simulink model "VisionModel_v7"  (Simulink 7.6)
settings: Solver=FixedStepDiscrete  StartTime=0.0  StopTime=0  RelTol=1e-3
values from neighbouring files (symbols this model uses):
  Down_Camera_Dimensions = [120 160]    [VisionConstants.m]
  Forward_Camera_Dimensions = [160 120]    [VisionConstants.m]
  Iter_Segment_Thresh = 60    [VisionConstants.m]
  Scale_Down_B = 1    [VisionConstants.m]
  Scale_Down_G = 1    [VisionConstants.m]
  Scale_Down_H = 1    [VisionConstants.m]
  Scale_Down_R = 1    [VisionConstants.m]
  Scale_Down_S = 1    [VisionConstants.m]
  Scale_Down_V = 5    [VisionConstants.m]
  Scale_Forward_B = 0    [VisionConstants.m]
  Scale_Forward_G = 1    [VisionConstants.m]
  Scale_Forward_H = 1    [VisionConstants.m]
  Scale_Forward_R = 0    [VisionConstants.m]
  Scale_Forward_S = 1    [VisionConstants.m]
  Scale_Forward_V = 5    [VisionConstants.m]
undefined symbols (not defined in the file or in its folder): Forward_Fov, Rec, SDTV
libraries: vipconversions x6, vipgeotforms x3, vipanalysis x2, viptransforms x2, viptextngfix x2
(part 1 of 2)
settings Model: Creator=Administrator  LastModifiedBy=auvt
settings OptimizationCC: OptimizeModelRefInitCode=on
settings RTWCC: SystemTargetFile=ert.tlc  GenCodeOnly=on  TemplateMakefile=ert_default_tmf  PostCodeGenCommand=packNGo(buildInfo, {'packType' 'flat'})  Description=Real-Time Workshop Embedded Coder  GenerateReport=on  ProcessScript=ert_make_rtw_hook  IncludeHyperlinkInReport=on  LaunchReport=on  TargetLang=C++
settings CodeAppCC: IgnoreCustomStorageClasses=off
settings ERTTargetCC: MultiwordLength=2048  GenerateSampleERTMain=on  IncludeMdlTerminateFcn=off  ERTCustomFileTemplate=example_file_process.tlc  ConvertIfToSwitch=off

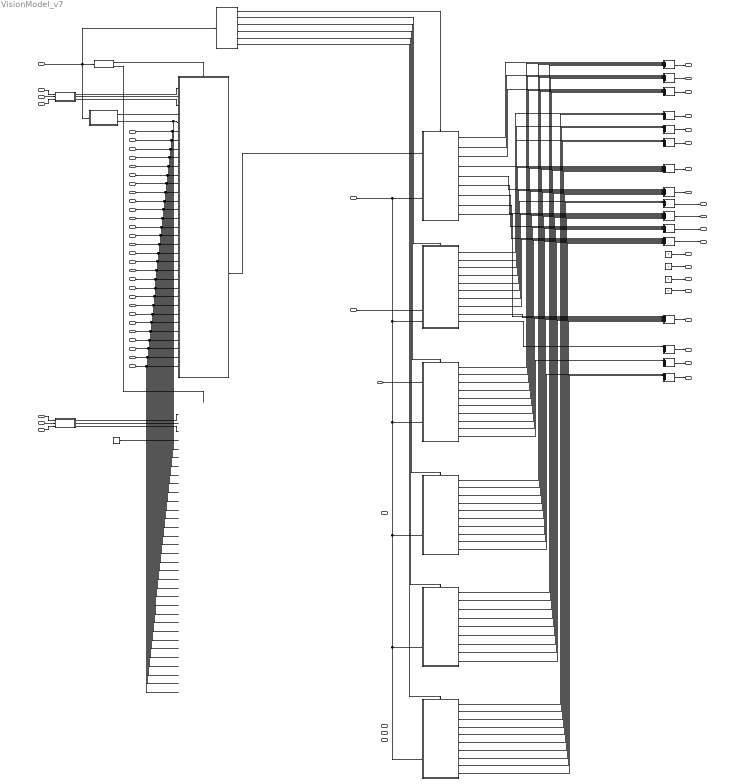
== system VisionModel_v7 ==
  note: Forward camera QImage array
  note: Down camera QImage array
  note: Forward
  note: Down
  note: Current target information
  note: Desired target information
  note: Mode and general target information
  note: Note: TargetFound, and the last three inputs to MotionController.mdl,
      | can be changed by the script, not the vision model.
  note: Path-following variables
      | DesiredPathDirection:
      | 0 = Use internal default
      | 1 = Take left path
      | 2 = Take right path
  note: Drop mechanism variables
  R_forward_in : Inport  PortDimensions=Forward_Camera_Dimensions
  G_forward_in : Inport  Port=2  PortDimensions=Forward_Camera_Dimensions
  B_forward_in : Inport  Port=3  PortDimensions=Forward_Camera_Dimensions
  R_down_in : Inport  Port=4  PortDimensions=Down_Camera_Dimensions
  G_down_in : Inport  Port=5  PortDimensions=Down_Camera_Dimensions
  B_down_in : Inport  Port=6  PortDimensions=Down_Camera_Dimensions
  ModeSelect : Inport  Port=7
  OutputImage : Inport  Port=8
  DesiredPathDirection : Inport  Port=9
  DesiredBuoyColor : Inport  Port=10
  DesiredTorpedoColor : Inport  Port=11
  ProceedToSecondTarget : Inport  Port=12
  DefaultTargetShape : Inport  Port=13
  DefaultTargetColor : Inport  Port=14
  white_al : Inport  Port=15
  white_au : Inport  Port=16
  white_bl : Inport  Port=17
  white_bu : Inport  Port=18
  black_al : Inport  Port=19
  black_au : Inport  Port=20
  black_bl : Inport  Port=21
  black_bu : Inport  Port=22
  blue_al : Inport  Port=23
  blue_au : Inport  Port=24
  blue_bl : Inport  Port=25
  blue_bu : Inport  Port=26
  red_al : Inport  Port=27
  red_au : Inport  Port=28
  red_bl : Inport  Port=29
  red_bu : Inport  Port=30
  orange_al : Inport  Port=31
  orane_au : Inport  Port=32
  orange_bl : Inport  Port=33
  orange_bu : Inport  Port=34
  yellow_al : Inport  Port=35
  yellow_au : Inport  Port=36
  yellow_bl : Inport  Port=37
  yellow_bu : Inport  Port=38
  green_al : Inport  Port=39
  green_au : Inport  Port=40
  breen_bl : Inport  Port=41
  green_bu : Inport  Port=42
  Add{,2..6,18..27} (16 alike) : Sum  Inputs=++++++
  Blob_Analysis : Subsystem  TreatAsAtomicUnit=on
  ColorSelect : Subsystem  TreatAsAtomicUnit=on
  Constant{,1..3} (4 alike) : Constant  Value=0
  Down Filter : Subsystem
  Forward Filter : Subsystem
  If1 : If  IfExpression=u1 == 1 | u1 == 3 | u1 == 4 | u1 == 5  ElseIfExpressions=u1 == 2 | u1 == 6  ShowElse=off
  If2 : If  IfExpression=u1 == 1  ElseIfExpressions=u1 == 2, u1 == 3, u1 == 4, u1 == 5, u1 == 6  ShowElse=off
  L_detector : Subsystem  TreatAsAtomicUnit=on
  ModeSelect1 : Constant  Value=[2 0 0 0 0 0 0 0 0 0]  SampleTime=-1
  buoy_detector : Subsystem  TreatAsAtomicUnit=on
  drop_mech : Subsystem  TreatAsAtomicUnit=on
  path_detector : Subsystem  TreatAsAtomicUnit=on
  torpedo : Subsystem  TreatAsAtomicUnit=on
  validation_gate : Subsystem  TreatAsAtomicUnit=on
  R_forward_out : Outport  OutDataTypeStr=double
  G_forward_out : Outport  Port=2  OutDataTypeStr=double
  B_forward_out : Outport  Port=3  OutDataTypeStr=double
  R_down_out : Outport  Port=4  OutDataTypeStr=double
  G_down_out : Outport  Port=5  OutDataTypeStr=double
  B_down_out : Outport  Port=6  OutDataTypeStr=double
  TargetSelect : Outport  Port=7  OutDataTypeStr=double
  MaintainHeading : Outport  Port=8  OutDataTypeStr=double
  TargetX : Outport  Port=9  OutDataTypeStr=double
  TargetY : Outport  Port=10  OutDataTypeStr=double
  TargetZ : Outport  Port=11  OutDataTypeStr=double
  TargetYaw : Outport  Port=12  OutDataTypeStr=double
  DesiredTargetX : Outport  Port=13  OutDataTypeStr=double
  DesiredTargetY : Outport  Port=14  OutDataTypeStr=double
  DesiredTargetZ : Outport  Port=15  OutDataTypeStr=double
  DesiredTargetYaw : Outport  Port=16  OutDataTypeStr=double
  TargetDetected : Outport  Port=17  OutDataTypeStr=double
  PathState : Outport  Port=18  OutDataTypeStr=double
  BuoyColors : Outport  Port=19  OutDataTypeStr=double
  FireAuthorization : Outport  Port=20  OutDataTypeStr=double
  wires:
  G_down_in/1 -> Down Filter/2(G_in)
  R_down_in/1 -> Down Filter/1(R_in)
  B_down_in/1 -> Down Filter/3(B_in)
  If1/1 -> Blob_Analysis/Action
  If1/2 -> ?
  R_forward_in/1 -> Forward Filter/1(R_in)
  Forward Filter/2(G_out) -> Blob_Analysis/2(G_in)
  Forward Filter/1(R_out) -> Blob_Analysis/1(R_in)
  Forward Filter/3(B_out) -> Blob_Analysis/3(B_in)
  G_forward_in/1 -> Forward Filter/2(G_in)
  B_forward_in/1 -> Forward Filter/3(B_in)
  Down Filter/2(G_out) -> ?
  Down Filter/1(R_out) -> ?
  Down Filter/3(B_out) -> ?
  Blob_Analysis/11(bw_image) -> validation_gate/1(bw_image)
  white_al/1 -> Blob_Analysis/6(white_al)
  white_au/1 -> Blob_Analysis/7(white_au)
  white_bl/1 -> Blob_Analysis/8(white_bl)
  white_bu/1 -> Blob_Analysis/9(white_bu)
  black_al/1 -> Blob_Analysis/10(black_al)
  black_au/1 -> Blob_Analysis/11(black_au)
  black_bl/1 -> Blob_Analysis/12(black_bl)
  black_bu/1 -> Blob_Analysis/13(black_bu)
  blue_al/1 -> Blob_Analysis/14(blue_al)
  blue_au/1 -> Blob_Analysis/15(blue_au)
  blue_bl/1 -> Blob_Analysis/16(blue_bl)
  blue_bu/1 -> Blob_Analysis/17(blue_bu)
  red_al/1 -> Blob_Analysis/18(red_al)
  red_au/1 -> Blob_Analysis/19(red_au)
  red_bl/1 -> Blob_Analysis/20(red_bl)
  red_bu/1 -> Blob_Analysis/21(red_bu)
  orange_al/1 -> Blob_Analysis/22(orange_al)
  orane_au/1 -> Blob_Analysis/23(orane_au)
  orange_bl/1 -> Blob_Analysis/24(orange_bl)
  orange_bu/1 -> Blob_Analysis/25(orange_bu)
  yellow_al/1 -> Blob_Analysis/26(yellow_al)
  yellow_au/1 -> Blob_Analysis/27(yellow_au)
  yellow_bl/1 -> Blob_Analysis/28(yellow_bl)
  yellow_bu/1 -> Blob_Analysis/29(yellow_bu)
  green_al/1 -> Blob_Analysis/30(green_al)
  green_au/1 -> Blob_Analysis/31(green_au)
  breen_bl/1 -> Blob_Analysis/32(breen_bl)
  green_bu/1 -> Blob_Analysis/33(green_bu)
  If2/1 -> validation_gate/Action
  Add2/1 -> MaintainHeading/1
  Add3/1 -> TargetX/1
  Add4/1 -> TargetY/1
  Add5/1 -> TargetZ/1
  Add6/1 -> TargetYaw/1
  Add19/1 -> PathState/1
  Add22/1 -> R_forward_out/1
  Add23/1 -> G_forward_out/1
  Add24/1 -> B_forward_out/1
  Constant/1 -> DesiredTargetX/1
  Constant3/1 -> DesiredTargetYaw/1
  Constant2/1 -> DesiredTargetZ/1
  Constant1/1 -> DesiredTargetY/1
  Add20/1 -> BuoyColors/1
  Add21/1 -> FireAuthorization/1
  validation_gate/1(R_forward_out) -> Add22/1
  validation_gate/2(G_forward_out) -> Add23/1
  validation_gate/3(B_forward_out) -> Add24/1
  validation_gate/4(TargetSelect) -> Add/1
  validation_gate/5(MaintainHeading) -> Add2/1
  validation_gate/6(TargetY) -> Add4/1
  validation_gate/7(TargetZ) -> Add5/1
  validation_gate/8(TargetYaw) -> Add6/1
  validation_gate/9(TargetDetected) -> Add18/1
  path_detector/1(R_down_out) -> Add25/1
  path_detector/2(G_down_out) -> Add26/1
  path_detector/3(B_down_out) -> Add27/1
  path_detector/4(TargetSelect) -> Add/2
  path_detector/5(MaintainHeading) -> Add2/2
  path_detector/6(TargetX) -> Add3/1
  path_detector/7(TargetY) -> Add4/2
  path_detector/8(TargetYaw) -> Add6/2
  path_detector/9(TargetDetected) -> Add18/2
  path_detector/10(PathState) -> Add19/1
  buoy_detector/1(R_forward_out) -> Add22/2
  buoy_detector/2(G_forward_out) -> Add23/2
  buoy_detector/3(B_forward_out) -> Add24/2
  buoy_detector/4(TargetSelect) -> Add/3
  buoy_detector/5(MaintainHeading) -> Add2/3
  buoy_detector/6(TargetY) -> Add4/3
  buoy_detector/7(TargetZ) -> Add5/2
  buoy_detector/8(TargetYaw) -> Add6/3
  buoy_detector/9(TargetDetected) -> Add18/3
  buoy_detector/10(BuoyColors) -> Add20/1
  torpedo/1(R_forward_out) -> Add22/3
  torpedo/2(G_forward_out) -> Add23/3
  torpedo/3(B_forward_out) -> Add24/3
  torpedo/4(TargetSelect) -> Add/4
  torpedo/5(MaintainHeading) -> Add2/4
  torpedo/6(TargetY) -> Add4/4
  torpedo/7(TargetZ) -> Add5/3
  torpedo/8(TargetYaw) -> Add6/4
  torpedo/10(FireAuthorization) -> Add21/1
  torpedo/9(TargetDetected) -> Add18/4
  L_detector/1(R_forward_out) -> Add22/4
  L_detector/2(G_forward_out) -> Add23/4
  L_detector/3(B_forward_out) -> Add24/4
  L_detector/4(TargetSelect) -> Add/5
  L_detector/5(MaintainHeading) -> Add2/5
  L_detector/6(TargetY) -> Add4/5
  L_detector/7(TargetZ) -> Add5/4
  L_detector/8(TargetYaw) -> Add6/5
  L_detector/9(TargetDetected) -> Add18/5
  drop_mech/1(R_down_out) -> Add25/2
  drop_mech/2(G_down_out) -> Add26/2
  drop_mech/3(B_down_out) -> Add27/2
  drop_mech/4(TargetSelect) -> Add/6
  drop_mech/5(MaintainHeading) -> Add2/6
  drop_mech/6(TargetX) -> Add3/2
  drop_mech/7(TargetY) -> Add4/6
  drop_mech/8(TargetYaw) -> Add6/6
  drop_mech/9(TargetDetected) -> Add18/6
  drop_mech/10(FireAuthorization) -> Add21/2
  ModeSelect/1 -> If1/1, ColorSelect/1(ModeSelect), If2/1
  If2/2 -> path_detector/Action
  If2/3 -> buoy_detector/Action
  If2/4 -> torpedo/Action
  If2/5 -> L_detector/Action
  If2/6 -> drop_mech/Action
  ColorSelect/1(ColorFilter) -> Blob_Analysis/4(ColorFilter)
  ColorSelect/2(OutputSegmentedImage) -> Blob_Analysis/5(OutputSegmentedImage)
  OutputImage/1 -> validation_gate/2(output_image), buoy_detector/2(output_image), torpedo/2(output_image), L_detector/2(output_image), drop_mech/2(output_image), path_detector/7(output_image)
  DesiredBuoyColor/1 -> buoy_detector/1(DesiredBuoyColor)
  DesiredPathDirection/1 -> path_detector/6(DesiredPathDirection)
  ? -> path_detector/1(bw_image)
  ? -> path_detector/2(blob_count)
  ? -> path_detector/3(blob_area)
  ? -> path_detector/4(blob_centroids)
  ? -> path_detector/5(blob_orientation)
  ModeSelect1/1 -> ?
  Add/1 -> TargetSelect/1
  Add25/1 -> R_down_out/1
  Add26/1 -> G_down_out/1
  Add27/1 -> B_down_out/1
  Add18/1 -> TargetDetected/1

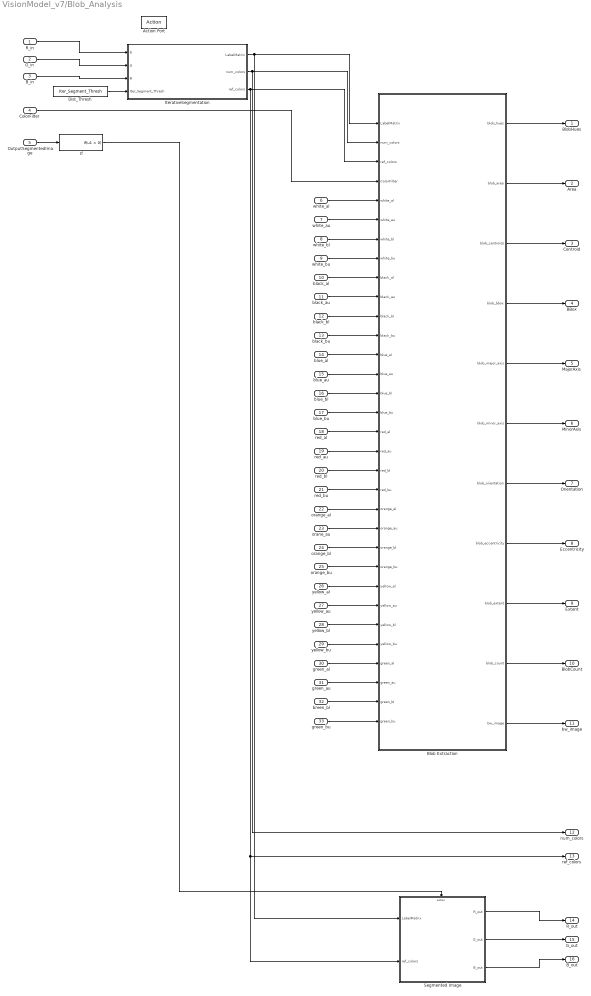
== system VisionModel_v7/Blob_Analysis ==
  R_in : Inport
  G_in : Inport  Port=2
  B_in : Inport  Port=3
  ColorFilter : Inport  Port=4
  OutputSegmentedImage : Inport  Port=5
  white_al : Inport  Port=6
  white_au : Inport  Port=7
  white_bl : Inport  Port=8
  white_bu : Inport  Port=9
  black_al : Inport  Port=10
  black_au : Inport  Port=11
  black_bl : Inport  Port=12
  black_bu : Inport  Port=13
  blue_al : Inport  Port=14
  blue_au : Inport  Port=15
  blue_bl : Inport  Port=16
  blue_bu : Inport  Port=17
  red_al : Inport  Port=18
  red_au : Inport  Port=19
  red_bl : Inport  Port=20
  red_bu : Inport  Port=21
  orange_al : Inport  Port=22
  orane_au : Inport  Port=23
  orange_bl : Inport  Port=24
  orange_bu : Inport  Port=25
  yellow_al : Inport  Port=26
  yellow_au : Inport  Port=27
  yellow_bl : Inport  Port=28
  yellow_bu : Inport  Port=29
  green_al : Inport  Port=30
  green_au : Inport  Port=31
  breen_bl : Inport  Port=32
  green_bu : Inport  Port=33
  Action Port : ActionPort  ActionType=then
  Blob Extraction : Stateflow chart  TreatAsAtomicUnit=on
  Dist_Thresh : Constant  Value=Iter_Segment_Thresh  SampleTime=-1
  If : If  ShowElse=off
  IterativeSegmentation : Subsystem
      settings: UndoDeleteFcn=Stateflow.SLINSF.SimulinkMan.restorePreDeleteFcn  PreDeleteFcn=Stateflow.SLINSF.SimulinkMan.removePreDeleteFcn
  Segmented Image : Subsystem  TreatAsAtomicUnit=on
  BlobHues : Outport
  Area : Outport  Port=2
  Centroid : Outport  Port=3
  BBox : Outport  Port=4
  MajorAxis : Outport  Port=5
  MinorAxis : Outport  Port=6
  Orientation : Outport  Port=7
  Eccentricity : Outport  Port=8
  Extent : Outport  Port=9
  BlobCount : Outport  Port=10
  bw_image : Outport  Port=11
  num_colors : Outport  Port=12
  ref_colors : Outport  Port=13
  R_out : Outport  Port=14
  G_out : Outport  Port=15
  B_out : Outport  Port=16
  wires:
  Blob Extraction/11(bw_image) -> bw_image/1
  Blob Extraction/10(blob_count) -> BlobCount/1
  Blob Extraction/9(blob_extent) -> Extent/1
  Blob Extraction/8(blob_eccentricity) -> Eccentricity/1
  Blob Extraction/7(blob_orientation) -> Orientation/1
  Blob Extraction/6(blob_minor_axis) -> MinorAxis/1
  Blob Extraction/5(blob_major_axis) -> MajorAxis/1
  Blob Extraction/4(blob_bbox) -> BBox/1
  Blob Extraction/3(blob_centroids) -> Centroid/1
  Blob Extraction/2(blob_area) -> Area/1
  Blob Extraction/1(blob_hues) -> BlobHues/1
  ColorFilter/1 -> Blob Extraction/4(ColorFilter)
  white_al/1 -> Blob Extraction/5(white_al)
  white_au/1 -> Blob Extraction/6(white_au)
  white_bl/1 -> Blob Extraction/7(white_bl)
  white_bu/1 -> Blob Extraction/8(white_bu)
  black_al/1 -> Blob Extraction/9(black_al)
  black_au/1 -> Blob Extraction/10(black_au)
  black_bl/1 -> Blob Extraction/11(black_bl)
  black_bu/1 -> Blob Extraction/12(black_bu)
  blue_au/1 -> Blob Extraction/14(blue_au)
  blue_bl/1 -> Blob Extraction/15(blue_bl)
  blue_bu/1 -> Blob Extraction/16(blue_bu)
  red_al/1 -> Blob Extraction/17(red_al)
  red_au/1 -> Blob Extraction/18(red_au)
  red_bl/1 -> Blob Extraction/19(red_bl)
  red_bu/1 -> Blob Extraction/20(red_bu)
  IterativeSegmentation/1(LabelMatrix) -> Blob Extraction/1(LabelMatrix), Segmented Image/1(LabelMatrix)
  IterativeSegmentation/2(num_colors) -> Blob Extraction/2(num_colors), num_colors/1
  IterativeSegmentation/3(ref_colors) -> Blob Extraction/3(ref_colors), Segmented Image/2(ref_colors), ref_colors/1
  Dist_Thresh/1 -> IterativeSegmentation/4(Iter_Segment_Thresh)
  R_in/1 -> IterativeSegmentation/1(R)
  G_in/1 -> IterativeSegmentation/2(G)
  B_in/1 -> IterativeSegmentation/3(B)
  If/1 -> Segmented Image/Action
  OutputSegmentedImage/1 -> If/1
  Segmented Image/1(R_out) -> R_out/1
  Segmented Image/2(G_out) -> G_out/1
  Segmented Image/3(B_out) -> B_out/1
  green_bu/1 -> Blob Extraction/32(green_bu)
  blue_al/1 -> Blob Extraction/13(blue_al)
  orange_al/1 -> Blob Extraction/21(orange_al)
  orane_au/1 -> Blob Extraction/22(orange_au)
  orange_bl/1 -> Blob Extraction/23(orange_bl)
  orange_bu/1 -> Blob Extraction/24(orange_bu)
  yellow_al/1 -> Blob Extraction/25(yellow_al)
  yellow_au/1 -> Blob Extraction/26(yellow_au)
  yellow_bl/1 -> Blob Extraction/27(yellow_bl)
  yellow_bu/1 -> Blob Extraction/28(yellow_bu)
  green_al/1 -> Blob Extraction/29(green_al)
  green_au/1 -> Blob Extraction/30(green_au)
  breen_bl/1 -> Blob Extraction/31(green_bl)

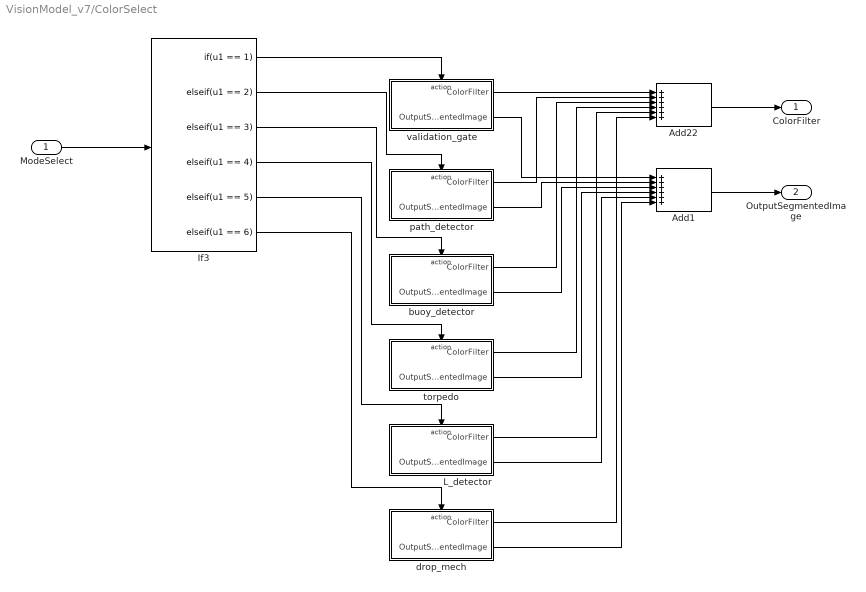
== system VisionModel_v7/ColorSelect ==
  ModeSelect : Inport
  Add1 : Sum  Inputs=++++++
  Add22 : Sum  Inputs=++++++
  If3 : If  IfExpression=u1 == 1  ElseIfExpressions=u1 == 2, u1 == 3, u1 == 4, u1 == 5, u1 == 6  ShowElse=off
  L_detector : Subsystem  TreatAsAtomicUnit=on
  buoy_detector : Subsystem  TreatAsAtomicUnit=on
  drop_mech : Subsystem  TreatAsAtomicUnit=on
  path_detector : Subsystem  TreatAsAtomicUnit=on
  torpedo : Subsystem  TreatAsAtomicUnit=on
  validation_gate : Subsystem  TreatAsAtomicUnit=on
  ColorFilter : Outport  OutDataTypeStr=double
  OutputSegmentedImage : Outport  Port=2  OutDataTypeStr=double
  wires:
  ModeSelect/1 -> If3/1
  If3/1 -> validation_gate/Action
  Add22/1 -> ColorFilter/1
  If3/2 -> path_detector/Action
  If3/3 -> buoy_detector/Action
  If3/4 -> torpedo/Action
  If3/5 -> L_detector/Action
  If3/6 -> drop_mech/Action
  Add1/1 -> OutputSegmentedImage/1
  validation_gate/1(ColorFilter) -> Add22/1
  validation_gate/2(OutputSegmentedImage) -> Add1/1
  path_detector/1(ColorFilter) -> Add22/2
  path_detector/2(OutputSegmentedImage) -> Add1/2
  buoy_detector/1(ColorFilter) -> Add22/3
  buoy_detector/2(OutputSegmentedImage) -> Add1/3
  torpedo/1(ColorFilter) -> Add22/4
  torpedo/2(OutputSegmentedImage) -> Add1/4
  L_detector/1(ColorFilter) -> Add22/5
  L_detector/2(OutputSegmentedImage) -> Add1/5
  drop_mech/1(ColorFilter) -> Add22/6
  drop_mech/2(OutputSegmentedImage) -> Add1/6

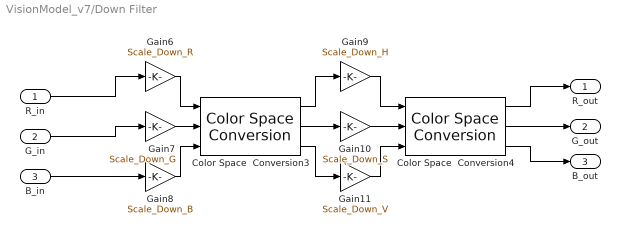
== system VisionModel_v7/Down Filter ==
  R_in : Inport  PortDimensions=Down_Camera_Dimensions
  G_in : Inport  Port=2  PortDimensions=Down_Camera_Dimensions
  B_in : Inport  Port=3  PortDimensions=Down_Camera_Dimensions
  Color Space  Conversion3 : vipconversions/Color Space  Conversion  conversion=Obsolete  conversionActive=R'G'B' to HSV  wp_str=D50  rec=Rec. 601 (SDTV)  sys=1125/60/2:1  imagePorts=Separate color signals
  Color Space  Conversion4 : vipconversions/Color Space  Conversion  conversion=Obsolete  conversionActive=HSV to R'G'B'  wp_str=D50  rec=Rec. 601 (SDTV)  sys=1125/60/2:1  imagePorts=Separate color signals
  Gain10 : Gain  Gain=Scale_Down_S
  Gain11 : Gain  Gain=Scale_Down_V
  Gain6 : Gain  Gain=Scale_Down_R
  Gain7 : Gain  Gain=Scale_Down_G
  Gain8 : Gain  Gain=Scale_Down_B
  Gain9 : Gain  Gain=Scale_Down_H
  R_out : Outport  OutDataTypeStr=double
  G_out : Outport  Port=2  OutDataTypeStr=double
  B_out : Outport  Port=3  OutDataTypeStr=double
  wires:
  Gain6/1 -> Color Space  Conversion3/1
  Gain7/1 -> Color Space  Conversion3/2
  Gain8/1 -> Color Space  Conversion3/3
  Color Space  Conversion3/1 -> Gain9/1
  Color Space  Conversion3/2 -> Gain10/1
  Color Space  Conversion3/3 -> Gain11/1
  Gain9/1 -> Color Space  Conversion4/1
  Gain10/1 -> Color Space  Conversion4/2
  Gain11/1 -> Color Space  Conversion4/3
  R_in/1 -> Gain6/1
  G_in/1 -> Gain7/1
  B_in/1 -> Gain8/1
  Color Space  Conversion4/1 -> R_out/1
  Color Space  Conversion4/2 -> G_out/1
  Color Space  Conversion4/3 -> B_out/1

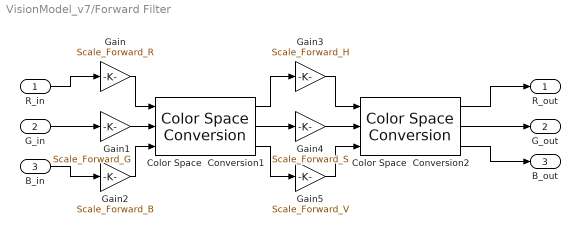
== system VisionModel_v7/Forward Filter ==
  R_in : Inport  PortDimensions=Forward_Camera_Dimensions
  G_in : Inport  Port=2  PortDimensions=Forward_Camera_Dimensions
  B_in : Inport  Port=3  PortDimensions=Forward_Camera_Dimensions
  Color Space  Conversion1 : vipconversions/Color Space  Conversion  conversion=Obsolete  conversionActive=R'G'B' to HSV  wp_str=D50  rec=Rec. 601 (SDTV)  sys=1125/60/2:1  imagePorts=Separate color signals
  Color Space  Conversion2 : vipconversions/Color Space  Conversion  conversion=Obsolete  conversionActive=HSV to R'G'B'  wp_str=D50  rec=Rec. 601 (SDTV)  sys=1125/60/2:1  imagePorts=Separate color signals
  Gain : Gain  Gain=Scale_Forward_R
  Gain1 : Gain  Gain=Scale_Forward_G
  Gain2 : Gain  Gain=Scale_Forward_B
  Gain3 : Gain  Gain=Scale_Forward_H
  Gain4 : Gain  Gain=Scale_Forward_S
  Gain5 : Gain  Gain=Scale_Forward_V
  R_out : Outport  OutDataTypeStr=double
  G_out : Outport  Port=2  OutDataTypeStr=double
  B_out : Outport  Port=3  OutDataTypeStr=double
  wires:
  R_in/1 -> Gain/1
  G_in/1 -> Gain1/1
  B_in/1 -> Gain2/1
  Gain/1 -> Color Space  Conversion1/1
  Gain1/1 -> Color Space  Conversion1/2
  Gain2/1 -> Color Space  Conversion1/3
  Color Space  Conversion1/1 -> Gain3/1
  Color Space  Conversion1/2 -> Gain4/1
  Color Space  Conversion1/3 -> Gain5/1
  Gain3/1 -> Color Space  Conversion2/1
  Gain4/1 -> Color Space  Conversion2/2
  Gain5/1 -> Color Space  Conversion2/3
  Color Space  Conversion2/1 -> R_out/1
  Color Space  Conversion2/2 -> G_out/1
  Color Space  Conversion2/3 -> B_out/1

== system VisionModel_v7/L_detector ==
  bw_image : Inport
  output_image : Inport  Port=2
  Action Port : ActionPort  ActionType=elseif
  R_forward_out : Outport  OutDataTypeStr=double
  G_forward_out : Outport  Port=2  OutDataTypeStr=double
  B_forward_out : Outport  Port=3  OutDataTypeStr=double
  TargetSelect : Outport  Port=4  OutDataTypeStr=double
  MaintainHeading : Outport  Port=5  OutDataTypeStr=double
  TargetY : Outport  Port=6  OutDataTypeStr=double
  TargetZ : Outport  Port=7  OutDataTypeStr=double
  TargetYaw : Outport  Port=8  OutDataTypeStr=double
  TargetDetected : Outport  Port=9  OutDataTypeStr=double

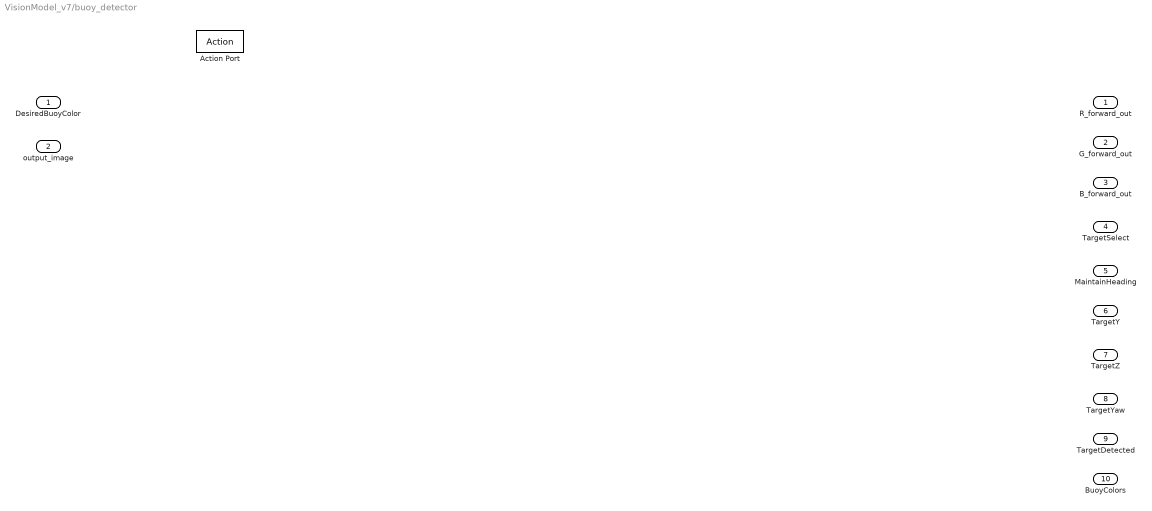
== system VisionModel_v7/buoy_detector ==
  DesiredBuoyColor : Inport
  output_image : Inport  Port=2
  Action Port : ActionPort  ActionType=elseif
  R_forward_out : Outport  OutDataTypeStr=double
  G_forward_out : Outport  Port=2  OutDataTypeStr=double
  B_forward_out : Outport  Port=3  OutDataTypeStr=double
  TargetSelect : Outport  Port=4  OutDataTypeStr=double
  MaintainHeading : Outport  Port=5  OutDataTypeStr=double
  TargetY : Outport  Port=6  OutDataTypeStr=double
  TargetZ : Outport  Port=7  OutDataTypeStr=double
  TargetYaw : Outport  Port=8  OutDataTypeStr=double
  TargetDetected : Outport  Port=9  OutDataTypeStr=double
  BuoyColors : Outport  Port=10  OutDataTypeStr=double

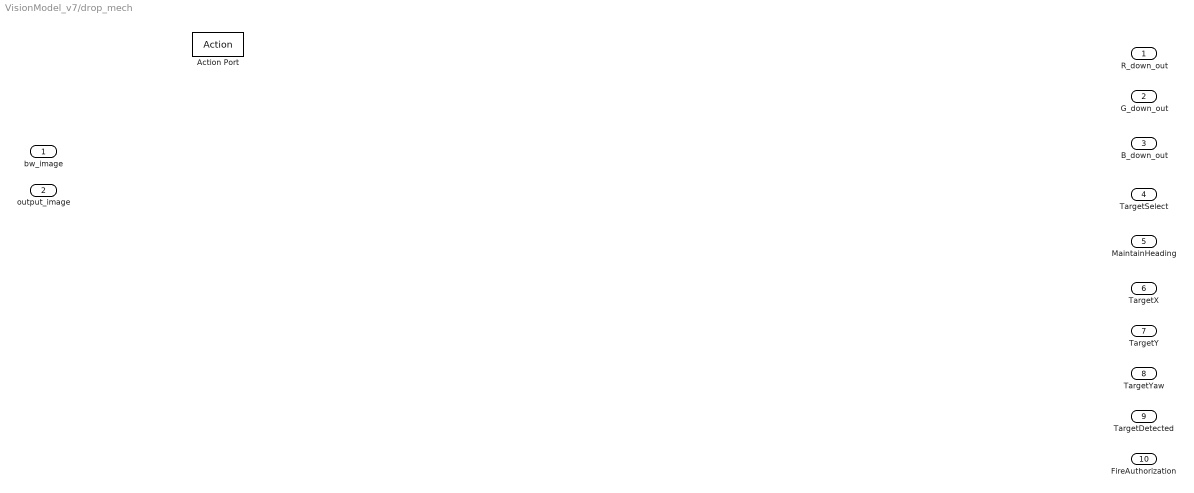
== system VisionModel_v7/drop_mech ==
  bw_image : Inport
  output_image : Inport  Port=2
  Action Port : ActionPort  ActionType=elseif
  R_down_out : Outport  OutDataTypeStr=double
  G_down_out : Outport  Port=2  OutDataTypeStr=double
  B_down_out : Outport  Port=3  OutDataTypeStr=double
  TargetSelect : Outport  Port=4  OutDataTypeStr=double
  MaintainHeading : Outport  Port=5  OutDataTypeStr=double
  TargetX : Outport  Port=6  OutDataTypeStr=double
  TargetY : Outport  Port=7  OutDataTypeStr=double
  TargetYaw : Outport  Port=8  OutDataTypeStr=double
  TargetDetected : Outport  Port=9  OutDataTypeStr=double
  FireAuthorization : Outport  Port=10  OutDataTypeStr=double

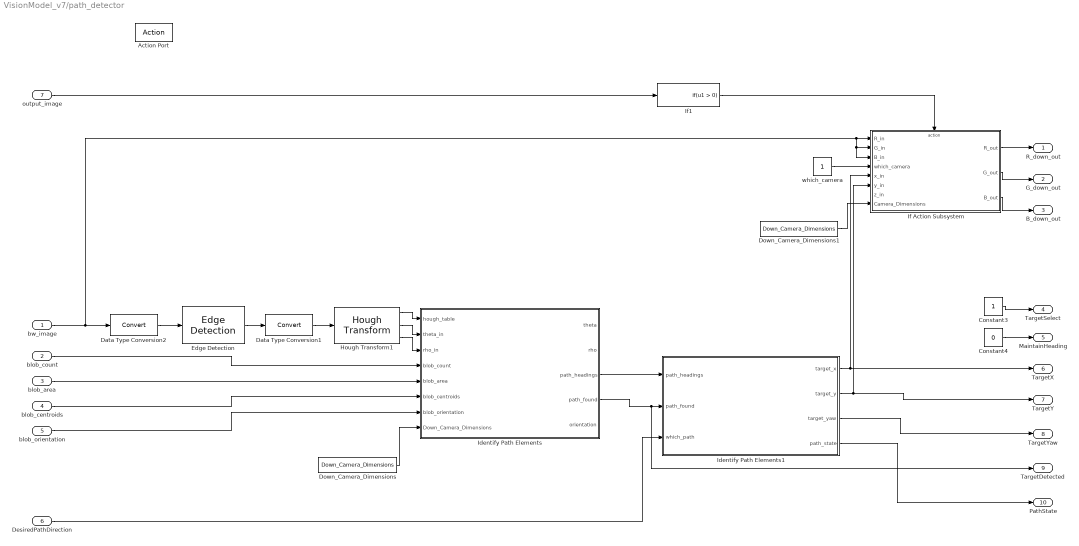
== system VisionModel_v7/path_detector ==
  bw_image : Inport
  blob_count : Inport  Port=2
  blob_area : Inport  Port=3
  blob_centroids : Inport  Port=4
  blob_orientation : Inport  Port=5
  DesiredPathDirection : Inport  Port=6
  output_image : Inport  Port=7
  Action Port : ActionPort  ActionType=elseif
  Constant3 : Constant  SampleTime=-1
  Constant4 : Constant  Value=0  SampleTime=-1
  Data Type Conversion1 : DataTypeConversion
  Data Type Conversion2 : DataTypeConversion
  Down_Camera_Dimensions : Constant  Value=Down_Camera_Dimensions  SampleTime=-1
  Down_Camera_Dimensions1 : Constant  Value=Down_Camera_Dimensions  SampleTime=-1
  Edge Detection : vipanalysis/Edge Detection  DialogController=vipDDGCreate  DialogControllerArgs=DataTag3  method=Sobel  outputType=Binary image  userDefinedThreshold=off  thresholdSource=Specify via dialog  threshold=20  thresholdTuning=3  edgeThinning=on  threshold_canny=[0.25 0.60]  autoPercent=70  sigma=1  roundingMode=Floor  overflowMode=off
  Hough Transform1 : viptransforms/Hough Transform  DialogController=vipDDGCreate  DialogControllerArgs=DataTag4  theta_res=pi/180  rho_res=1  out_theta_rho=on  outdtmode=double  firstCoeffMode=Binary point scaling  firstCoeffWordLength=16  firstCoeffFracLength=14  secondCoeffMode=Binary point scaling  secondCoeffWordLength=32  secondCoeffFracLength=16  outputMode=Binary point scaling  outputWordLength=16  outputFracLength=0  accumMode=Binary point scaling  accumWordLength=32  accumFracLength=20  prodOutputMode=Binary point scaling  prodOutputWordLength=32  prodOutputFracLength=20  memoryMode=Binary point scaling  memoryWordLength=32  memoryFracLength=16  roundingMode=Nearest  overflowMode=on
  Identify Path Elements : Stateflow chart  TreatAsAtomicUnit=on  SystemSampleTime=[1/30 0]
  Identify Path Elements1 : Stateflow chart  TreatAsAtomicUnit=on  SystemSampleTime=[1/30 0]
  If Action Subsystem : Subsystem  TreatAsAtomicUnit=on
  If1 : If  ShowElse=off
  which_camera : Constant  SampleTime=-1
  R_down_out : Outport  OutDataTypeStr=double
  G_down_out : Outport  Port=2  OutDataTypeStr=double
  B_down_out : Outport  Port=3  OutDataTypeStr=double
  TargetSelect : Outport  Port=4  OutDataTypeStr=double
  MaintainHeading : Outport  Port=5  OutDataTypeStr=double
  TargetX : Outport  Port=6  OutDataTypeStr=double
  TargetY : Outport  Port=7  OutDataTypeStr=double
  TargetYaw : Outport  Port=8  OutDataTypeStr=double
  TargetDetected : Outport  Port=9  OutDataTypeStr=double
  PathState : Outport  Port=10  OutDataTypeStr=double
  wires:
  Data Type Conversion2/1 -> Edge Detection/1
  bw_image/1 -> Data Type Conversion2/1, If Action Subsystem/1(R_in), If Action Subsystem/2(G_in), If Action Subsystem/3(B_in)
  Edge Detection/1 -> Data Type Conversion1/1
  Data Type Conversion1/1 -> Hough Transform1/1
  Hough Transform1/1 -> Identify Path Elements/1(hough_table)
  Hough Transform1/2 -> Identify Path Elements/2(theta_in)
  Hough Transform1/3 -> Identify Path Elements/3(rho_in)
  Down_Camera_Dimensions/1 -> Identify Path Elements/8(Down_Camera_Dimensions)
  blob_count/1 -> Identify Path Elements/4(blob_count)
  blob_area/1 -> Identify Path Elements/5(blob_area)
  blob_centroids/1 -> Identify Path Elements/6(blob_centroids)
  blob_orientation/1 -> Identify Path Elements/7(blob_orientation)
  Identify Path Elements/3(path_headings) -> Identify Path Elements1/1(path_headings)
  Identify Path Elements/4(path_found) -> Identify Path Elements1/2(path_found), TargetDetected/1
  DesiredPathDirection/1 -> Identify Path Elements1/3(which_path)
  Identify Path Elements1/1(target_x) -> TargetX/1, If Action Subsystem/5(x_in)
  Identify Path Elements1/2(target_y) -> TargetY/1, If Action Subsystem/6(y_in)
  Identify Path Elements1/3(target_yaw) -> TargetYaw/1
  Identify Path Elements1/4(path_state) -> PathState/1
  Constant3/1 -> TargetSelect/1
  Constant4/1 -> MaintainHeading/1
  If1/1 -> If Action Subsystem/Action
  output_image/1 -> If1/1
  which_camera/1 -> If Action Subsystem/4(which_camera)
  Down_Camera_Dimensions1/1 -> If Action Subsystem/8(Camera_Dimensions)
  If Action Subsystem/1(R_out) -> R_down_out/1
  If Action Subsystem/2(G_out) -> G_down_out/1
  If Action Subsystem/3(B_out) -> B_down_out/1

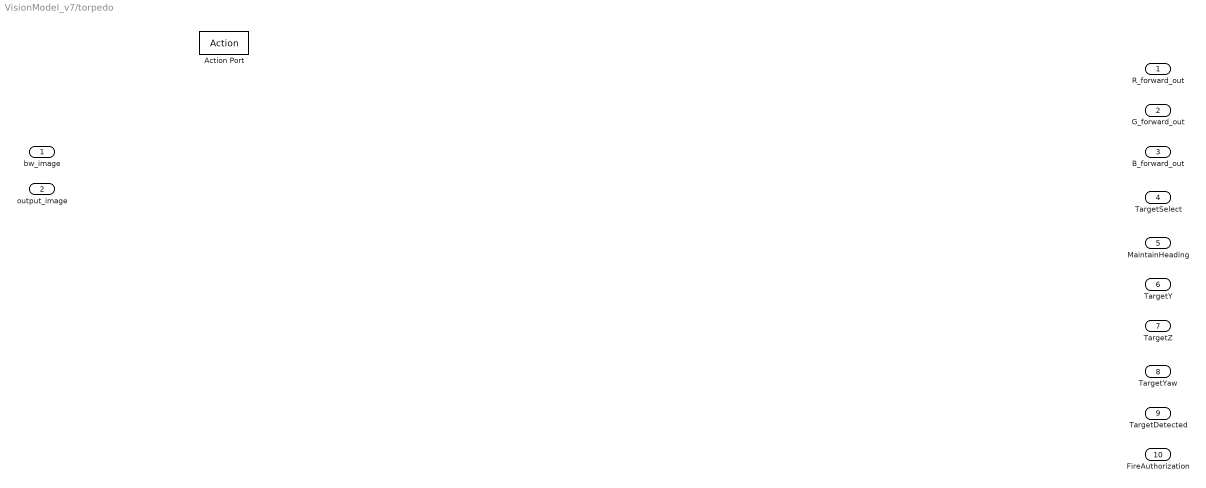
== system VisionModel_v7/torpedo ==
  bw_image : Inport
  output_image : Inport  Port=2
  Action Port : ActionPort  ActionType=elseif
  R_forward_out : Outport  OutDataTypeStr=double
  G_forward_out : Outport  Port=2  OutDataTypeStr=double
  B_forward_out : Outport  Port=3  OutDataTypeStr=double
  TargetSelect : Outport  Port=4  OutDataTypeStr=double
  MaintainHeading : Outport  Port=5  OutDataTypeStr=double
  TargetY : Outport  Port=6  OutDataTypeStr=double
  TargetZ : Outport  Port=7  OutDataTypeStr=double
  TargetYaw : Outport  Port=8  OutDataTypeStr=double
  TargetDetected : Outport  Port=9  OutDataTypeStr=double
  FireAuthorization : Outport  Port=10  OutDataTypeStr=double

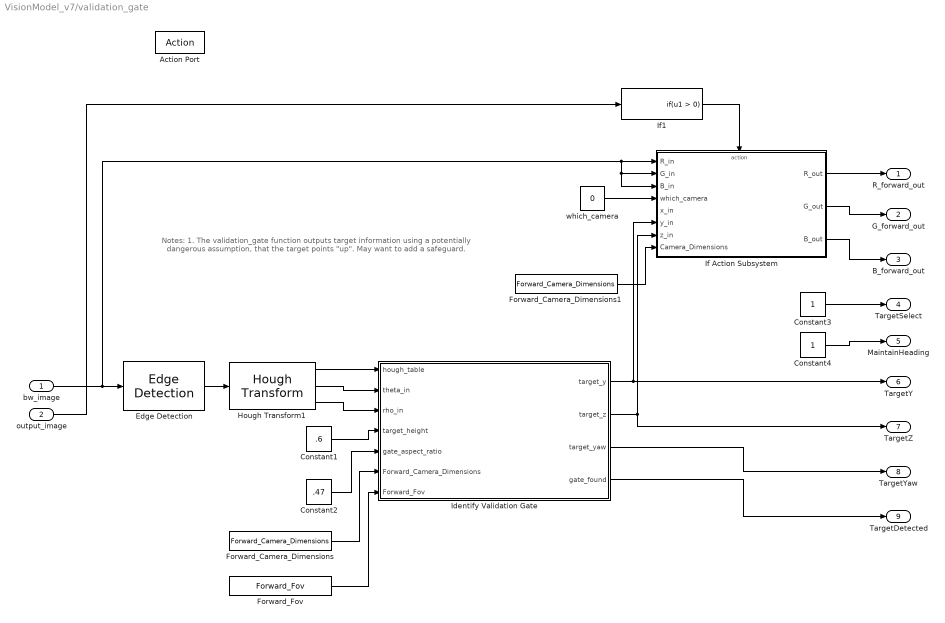
== system VisionModel_v7/validation_gate ==
  note: Notes:
      | 1. The validation_gate function outputs target
      | information using a potentially dangerous
      | assumption, that the target points "up". May
      | want to add a safeguard.
  bw_image : Inport  PortDimensions=Forward_Camera_Dimensions
  output_image : Inport  Port=2
  Action Port : ActionPort  ActionType=then
  Constant1 : Constant  Value=.6  SampleTime=-1
  Constant2 : Constant  Value=.47  SampleTime=-1
  Constant3 : Constant  SampleTime=-1
  Constant4 : Constant  SampleTime=-1
  Edge Detection : vipanalysis/Edge Detection  DialogController=vipDDGCreate  DialogControllerArgs=DataTag6  method=Sobel  outputType=Binary image  userDefinedThreshold=off  thresholdSource=Specify via dialog  threshold=0  thresholdTuning=3  edgeThinning=on  threshold_canny=[0.25 0.60]  autoPercent=70  sigma=1  roundingMode=Floor  overflowMode=off
  Forward_Camera_Dimensions : Constant  Value=Forward_Camera_Dimensions  SampleTime=-1
  Forward_Camera_Dimensions1 : Constant  Value=Forward_Camera_Dimensions  SampleTime=-1
  Forward_Fov : Constant  Value=Forward_Fov  SampleTime=-1
  Hough Transform1 : viptransforms/Hough Transform  DialogController=vipDDGCreate  DialogControllerArgs=DataTag7  theta_res=pi/180  rho_res=1  out_theta_rho=on  outdtmode=double  firstCoeffMode=Binary point scaling  firstCoeffWordLength=16  firstCoeffFracLength=14  secondCoeffMode=Binary point scaling  secondCoeffWordLength=32  secondCoeffFracLength=16  outputMode=Binary point scaling  outputWordLength=16  outputFracLength=0  accumMode=Binary point scaling  accumWordLength=32  accumFracLength=20  prodOutputMode=Binary point scaling  prodOutputWordLength=32  prodOutputFracLength=20  memoryMode=Binary point scaling  memoryWordLength=32  memoryFracLength=16  roundingMode=Nearest  overflowMode=on
  Identify Validation Gate : Stateflow chart  TreatAsAtomicUnit=on
  If Action Subsystem : Subsystem  TreatAsAtomicUnit=on
  If1 : If  ShowElse=off
  which_camera : Constant  Value=0  SampleTime=-1
  R_forward_out : Outport  OutDataTypeStr=double
  G_forward_out : Outport  Port=2  OutDataTypeStr=double
  B_forward_out : Outport  Port=3  OutDataTypeStr=double
  TargetSelect : Outport  Port=4  OutDataTypeStr=double
  MaintainHeading : Outport  Port=5  OutDataTypeStr=double
  TargetY : Outport  Port=6  OutDataTypeStr=double
  TargetZ : Outport  Port=7  OutDataTypeStr=double
  TargetYaw : Outport  Port=8  OutDataTypeStr=double
  TargetDetected : Outport  Port=9  OutDataTypeStr=double
  wires:
  Constant1/1 -> Identify Validation Gate/4(target_height)
  Constant2/1 -> Identify Validation Gate/5(gate_aspect_ratio)
  Forward_Camera_Dimensions/1 -> Identify Validation Gate/6(Forward_Camera_Dimensions)
  Forward_Fov/1 -> Identify Validation Gate/7(Forward_Fov)
  Identify Validation Gate/1(target_y) -> If Action Subsystem/6(y_in), TargetY/1
  Identify Validation Gate/2(target_z) -> If Action Subsystem/7(z_in), TargetZ/1
  If1/1 -> If Action Subsystem/Action
  which_camera/1 -> If Action Subsystem/4(which_camera)
  output_image/1 -> If1/1
  bw_image/1 -> If Action Subsystem/1(R_in), If Action Subsystem/2(G_in), If Action Subsystem/3(B_in), Edge Detection/1
  Forward_Camera_Dimensions1/1 -> If Action Subsystem/8(Camera_Dimensions)
  Hough Transform1/1 -> Identify Validation Gate/1(hough_table)
  Hough Transform1/2 -> Identify Validation Gate/2(theta_in)
  Hough Transform1/3 -> Identify Validation Gate/3(rho_in)
  Edge Detection/1 -> Hough Transform1/1
  If Action Subsystem/1(R_out) -> R_forward_out/1
  If Action Subsystem/2(G_out) -> G_forward_out/1
  If Action Subsystem/3(B_out) -> B_forward_out/1
  Constant3/1 -> TargetSelect/1
  Constant4/1 -> MaintainHeading/1
  Identify Validation Gate/3(target_yaw) -> TargetYaw/1
  Identify Validation Gate/4(gate_found) -> TargetDetected/1

== system VisionModel_v7/Blob_Analysis/IterativeSegmentation ==
  R : Inport
  G : Inport  Port=2
  B : Inport  Port=3
  Iter_Segment_Thresh : Inport  Port=4
  Color Space  Conversion1 : vipconversions/Color Space  Conversion  conversion=Obsolete  conversionActive=sR'G'B' to L*a*b*  wp_str=D50  rec=Rec. 601 (SDTV)  sys=1125/60/2:1  imagePorts=Separate color signals
  Low Pass Filter : Subsystem
  Segmentation : Subsystem
  LabelMatrix : Outport
  num_colors : Outport  Port=2
  ref_colors : Outport  Port=3
  wires:
  Low Pass Filter/3(B') -> Color Space  Conversion1/3
  Low Pass Filter/2(G') -> Color Space  Conversion1/2
  Low Pass Filter/1(R') -> Color Space  Conversion1/1
  Color Space  Conversion1/3 -> Segmentation/3(b)
  Color Space  Conversion1/2 -> Segmentation/2(a)
  Color Space  Conversion1/1 -> Segmentation/1(L)
  R/1 -> Low Pass Filter/1(R)
  G/1 -> Low Pass Filter/2(G)
  B/1 -> Low Pass Filter/3(B)
  Segmentation/1(LabelMatrix) -> LabelMatrix/1
  Segmentation/2(num_colors) -> num_colors/1
  Segmentation/3(ref_colors) -> ref_colors/1
  Iter_Segment_Thresh/1 -> Segmentation/4(Iter_Segment_Thresh)

== system VisionModel_v7/Blob_Analysis/Segmented Image ==
  LabelMatrix : Inport
  ref_colors : Inport  Port=2
  Action Port : ActionPort  ActionType=then
  Color Space  Conversion : vipconversions/Color Space  Conversion  conversion=Obsolete  conversionActive=L*a*b* to sR'G'B'  wp_str=D65  rec=Rec. 601 (SDTV)  sys=1125/60/2:1  imagePorts=Separate color signals
  Display Image : Stateflow chart  TreatAsAtomicUnit=on
  R_out : Outport
  G_out : Outport  Port=2
  B_out : Outport  Port=3
  wires:
  LabelMatrix/1 -> Display Image/1(LabelMatrix)
  ref_colors/1 -> Display Image/2(ref_colors)
  Display Image/1(L) -> Color Space  Conversion/1
  Display Image/2(a) -> Color Space  Conversion/2
  Display Image/3(b) -> Color Space  Conversion/3
  Color Space  Conversion/1 -> R_out/1
  Color Space  Conversion/2 -> G_out/1
  Color Space  Conversion/3 -> B_out/1

== system VisionModel_v7/ColorSelect/L_detector ==
  Action Port : ActionPort  ActionType=elseif
  ColorFilter1 : Constant  Value=[7 0 0 0 0 0 0 0 0 0]  SampleTime=-1
  OutputSegmentedImage1 : Constant  Value=0  SampleTime=-1
  ColorFilter : Outport  OutDataTypeStr=double
  OutputSegmentedImage : Outport  Port=2  OutDataTypeStr=double
  wires:
  ColorFilter1/1 -> ColorFilter/1
  OutputSegmentedImage1/1 -> OutputSegmentedImage/1

== system VisionModel_v7/ColorSelect/buoy_detector ==
  Action Port : ActionPort  ActionType=elseif
  ColorFilter1 : Constant  Value=[3 4 5 6 7 0 0 0 0 0]  SampleTime=-1
  OutputSegmentedImage1 : Constant  Value=0  SampleTime=-1
  ColorFilter : Outport  OutDataTypeStr=double
  OutputSegmentedImage : Outport  Port=2  OutDataTypeStr=double
  wires:
  ColorFilter1/1 -> ColorFilter/1
  OutputSegmentedImage1/1 -> OutputSegmentedImage/1

== system VisionModel_v7/ColorSelect/drop_mech ==
  Action Port : ActionPort  ActionType=elseif
  ColorFilter1 : Constant  Value=[1 2 4 0 0 0 0 0 0 0]  SampleTime=-1
  OutputSegmentedImage1 : Constant  Value=0  SampleTime=-1
  ColorFilter : Outport  OutDataTypeStr=double
  OutputSegmentedImage : Outport  Port=2  OutDataTypeStr=double
  wires:
  OutputSegmentedImage1/1 -> OutputSegmentedImage/1
  ColorFilter1/1 -> ColorFilter/1

== system VisionModel_v7/ColorSelect/path_detector ==
  Action Port : ActionPort  ActionType=elseif
  ColorFilter1 : Constant  Value=[5 6 0 0 0 0 0 0 0 0]  SampleTime=-1
  OutputSegmentedImage1 : Constant  Value=0  SampleTime=-1
  ColorFilter : Outport  OutDataTypeStr=double
  OutputSegmentedImage : Outport  Port=2  OutDataTypeStr=double
  wires:
  OutputSegmentedImage1/1 -> OutputSegmentedImage/1
  ColorFilter1/1 -> ColorFilter/1

== system VisionModel_v7/ColorSelect/torpedo ==
  Action Port : ActionPort  ActionType=elseif
  ColorFilter1 : Constant  Value=[3 4 0 0 0 0 0 0 0 0]  SampleTime=-1
  OutputSegmentedImage1 : Constant  Value=0  SampleTime=-1
  ColorFilter : Outport  OutDataTypeStr=double
  OutputSegmentedImage : Outport  Port=2  OutDataTypeStr=double
  wires:
  OutputSegmentedImage1/1 -> OutputSegmentedImage/1
  ColorFilter1/1 -> ColorFilter/1

== system VisionModel_v7/ColorSelect/validation_gate ==
  Action Port : ActionPort  ActionType=then
  ColorFilter1 : Constant  Value=[1 5 0 0 0 0 0 0 0 0]  SampleTime=-1
  OutputSegmentedImage1 : Constant  Value=0  SampleTime=-1
  ColorFilter : Outport  OutDataTypeStr=double
  OutputSegmentedImage : Outport  Port=2  OutDataTypeStr=double
  wires:
  ColorFilter1/1 -> ColorFilter/1
  OutputSegmentedImage1/1 -> OutputSegmentedImage/1

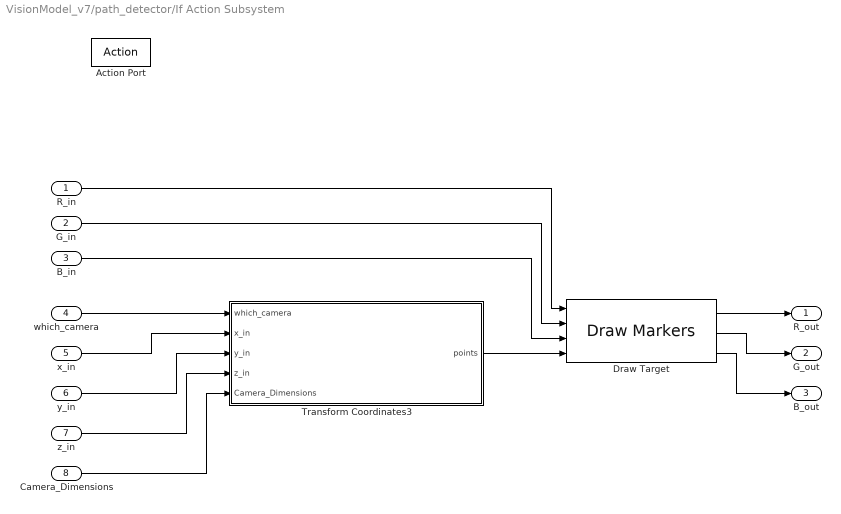
== system VisionModel_v7/path_detector/If Action Subsystem ==
  R_in : Inport
  G_in : Inport  Port=2
  B_in : Inport  Port=3
  which_camera : Inport  Port=4
  x_in : Inport  Port=5
  y_in : Inport  Port=6
  z_in : Inport  Port=7
  Camera_Dimensions : Inport  Port=8
  Action Port : ActionPort  ActionType=then
  Draw Target : viptextngfix/Draw Markers  DialogController=vipDDGCreate  DialogControllerArgs=DataTag5  shape=X-mark  size=7  fill=off  fillClrSource=Specify via dialog  display=User-specified value  intensity=200  color=[1 0 0]  opacity=0.6  viewport=Entire image  antialiasing=off  inType=Obsolete  imagePorts=Separate color signals  prodOutputMode=Binary point scaling  prodOutputWordLength=32  prodOutputFracLength=14  memoryMode=Specify word length  memoryWordLength=16  memoryFracLength=15  roundingMode=Floor  overflowMode=off
  Transform Coordinates3 : Stateflow chart  TreatAsAtomicUnit=on
  R_out : Outport  OutDataTypeStr=double
  G_out : Outport  Port=2  OutDataTypeStr=double
  B_out : Outport  Port=3  OutDataTypeStr=double
  wires:
  which_camera/1 -> Transform Coordinates3/1(which_camera)
  x_in/1 -> Transform Coordinates3/2(x_in)
  y_in/1 -> Transform Coordinates3/3(y_in)
  z_in/1 -> Transform Coordinates3/4(z_in)
  Camera_Dimensions/1 -> Transform Coordinates3/5(Camera_Dimensions)
  Draw Target/1 -> R_out/1
  Transform Coordinates3/1(points) -> Draw Target/4
  Draw Target/2 -> G_out/1
  Draw Target/3 -> B_out/1
  R_in/1 -> Draw Target/1
  G_in/1 -> Draw Target/2
  B_in/1 -> Draw Target/3

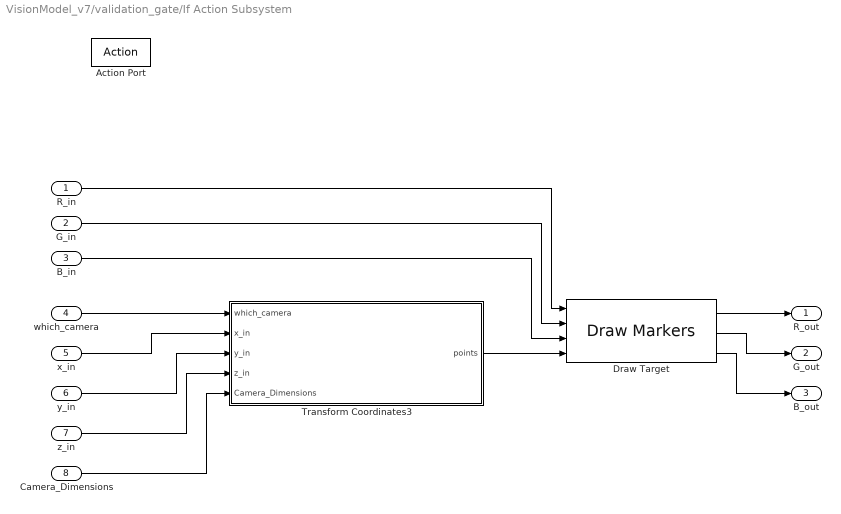
== system VisionModel_v7/validation_gate/If Action Subsystem ==
  R_in : Inport
  G_in : Inport  Port=2
  B_in : Inport  Port=3
  which_camera : Inport  Port=4
  x_in : Inport  Port=5
  y_in : Inport  Port=6
  z_in : Inport  Port=7
  Camera_Dimensions : Inport  Port=8
  Action Port : ActionPort  ActionType=then
  Draw Target : viptextngfix/Draw Markers  DialogController=vipDDGCreate  DialogControllerArgs=DataTag8  shape=X-mark  size=7  fill=off  fillClrSource=Specify via dialog  display=User-specified value  intensity=200  color=[1 0 0]  opacity=0.6  viewport=Entire image  antialiasing=off  inType=Obsolete  imagePorts=Separate color signals  prodOutputMode=Binary point scaling  prodOutputWordLength=32  prodOutputFracLength=14  memoryMode=Specify word length  memoryWordLength=16  memoryFracLength=15  roundingMode=Floor  overflowMode=off
  Transform Coordinates3 : Stateflow chart  TreatAsAtomicUnit=on
  R_out : Outport  OutDataTypeStr=double
  G_out : Outport  Port=2  OutDataTypeStr=double
  B_out : Outport  Port=3  OutDataTypeStr=double
  wires:
  which_camera/1 -> Transform Coordinates3/1(which_camera)
  x_in/1 -> Transform Coordinates3/2(x_in)
  y_in/1 -> Transform Coordinates3/3(y_in)
  z_in/1 -> Transform Coordinates3/4(z_in)
  Camera_Dimensions/1 -> Transform Coordinates3/5(Camera_Dimensions)
  Draw Target/1 -> R_out/1
  Transform Coordinates3/1(points) -> Draw Target/4
  Draw Target/2 -> G_out/1
  Draw Target/3 -> B_out/1
  R_in/1 -> Draw Target/1
  G_in/1 -> Draw Target/2
  B_in/1 -> Draw Target/3

== system VisionModel_v7/Blob_Analysis/IterativeSegmentation/Low Pass Filter ==
  R : Inport
  G : Inport  Port=2
  B : Inport  Port=3
  Low Pass Filter : Stateflow chart  TreatAsAtomicUnit=on
  Low Pass Filter1 : Stateflow chart  TreatAsAtomicUnit=on
  Low Pass Filter2 : Stateflow chart  TreatAsAtomicUnit=on
  R' : Outport
  G' : Outport  Port=2
  B' : Outport  Port=3
  wires:
  Low Pass Filter/1(Iout) -> R'/1
  Low Pass Filter2/1(Iout) -> B'/1
  Low Pass Filter1/1(Iout) -> G'/1
  B/1 -> Low Pass Filter2/1(I)
  G/1 -> Low Pass Filter1/1(I)
  R/1 -> Low Pass Filter/1(I)

== system VisionModel_v7/Blob_Analysis/IterativeSegmentation/Segmentation ==
  L : Inport
  a : Inport  Port=2
  b : Inport  Port=3
  Iter_Segment_Thresh : Inport  Port=4
  LabSegmentation : Stateflow chart  TreatAsAtomicUnit=on
  Reference Color Selection : Stateflow chart  TreatAsAtomicUnit=on
  Resize : Subsystem
  LabelMatrix : Outport
  num_colors : Outport  Port=2
  ref_colors : Outport  Port=3
  wires:
  Iter_Segment_Thresh/1 -> Reference Color Selection/4(Dist_Thresh)
  LabSegmentation/1(LabelMatrix) -> LabelMatrix/1
  Reference Color Selection/2(num_colors) -> LabSegmentation/5(num_colors), num_colors/1
  Reference Color Selection/1(ref_colors) -> ref_colors/1, LabSegmentation/4(ref_colors)
  Resize/3(Out3) -> Reference Color Selection/3(b)
  Resize/2(Out2) -> Reference Color Selection/2(a)
  Resize/1(Out1) -> Reference Color Selection/1(L)
  b/1 -> LabSegmentation/3(b), Resize/3(In3)
  a/1 -> LabSegmentation/2(a), Resize/2(In2)
  L/1 -> LabSegmentation/1(L), Resize/1(In1)

== system VisionModel_v7/Blob_Analysis/IterativeSegmentation/Segmentation/Resize ==
  In1 : Inport
  In2 : Inport  Port=2
  In3 : Inport  Port=3
  Resize : vipgeotforms/Resize  DialogController=vipDDGCreate  DialogControllerArgs=DataTag0  specify=Number of output rows and columns  rfactor=[]  outCols=25  outRows=25  outRowsCols=[60 80]  interp_method=Bilinear  antialias=on  useROI=off  roiFlag=off  prodOutputMode=Binary point scaling  prodOutputWordLength=32  prodOutputFracLength=10  roundingMode=Nearest  overflowMode=on
  Resize1 : vipgeotforms/Resize  DialogController=vipDDGCreate  DialogControllerArgs=DataTag1  specify=Number of output rows and columns  rfactor=[200 150]  outCols=25  outRows=25  outRowsCols=[60 80]  interp_method=Bilinear  antialias=on  useROI=off  roiFlag=off  prodOutputMode=Binary point scaling  prodOutputWordLength=32  prodOutputFracLength=10  roundingMode=Nearest  overflowMode=on
  Resize2 : vipgeotforms/Resize  DialogController=vipDDGCreate  DialogControllerArgs=DataTag2  specify=Number of output rows and columns  rfactor=[200 150]  outCols=25  outRows=25  outRowsCols=[60 80]  interp_method=Bilinear  antialias=on  useROI=off  roiFlag=off  prodOutputMode=Binary point scaling  prodOutputWordLength=32  prodOutputFracLength=10  roundingMode=Nearest  overflowMode=on
  Out1 : Outport
  Out2 : Outport  Port=2
  Out3 : Outport  Port=3
  wires:
  Resize2/1 -> Out3/1
  In3/1 -> Resize2/1
  Resize1/1 -> Out2/1
  In2/1 -> Resize1/1
  Resize/1 -> Out1/1
  In1/1 -> Resize/1

== matlab function validation_gate/Identify Validation Gate ==
  data: hough_table input double; target_y output double; target_z output double; target_yaw output double; gate_found output double; theta_in input double; rho_in input double; target_height input double; gate_aspect_ratio input double; Forward_Camera_Dimensions input double; Forward_Fov input double
function [target_y, target_z, target_yaw, gate_found] = validation_gate(hough_table, theta_in, rho_in, target_height, gate_aspect_ratio, Forward_Camera_Dimensions, Forward_Fov)
%#eml



% This function attempts to identfiy the validation gate, and returns
%   targeting information, and a true/false gate_found parameter.
%
% 5-29-11
%
% Input
%
%   target_height = fraction of goal post height to aim AUV at
%   gate_aspect_ratio = used to infer unknown points with little extra
%     processing (height/width of large goalpost-shape)
%
% Output
%
% Notes:
%   The hough_table is destroyed in this function (acceptable if
%     hough_table is not an output)
%   Process:
%     1. Identify primary, relatively "long" lines
%     2. 


%% Initialize
% Only the (max_num_lines) with the most votes will be considered as
%   candidates for the validation gate
max_num_lines = 200;
[rho_length, theta_length] = size(hough_table);
%rows = Forward_Camera_Dimensions(1);
%cols = Forward_Camera_Dimensions(2);
rows = 160;
cols = 120;


% eps_rho must be at least as big as the gate leg diameter (units of
%   pixels)
eps_rho = .1*max(rows,cols);
% eps_theta is used to distinguish lines as "horizontal" or "vertical";
%   units are radians
eps_theta = 10*pi/180;


% These vectors contain the final three lines that compose the validation gate
rho_gate = zeros(1,3);
theta_gate = zeros(1,3);

% These vectors contain intermediate line information; as lines are
%   eliminated from these vectors, their values are set to zero
rho = zeros(1,max_num_lines);
theta = zeros(1,max_num_lines);





% Identify the most popular max_num_lines lines
i_index = ones(1,max_num_lines);
j_index = ones(1,max_num_lines);

m = 1;
while( m <= max_num_lines )
    
    max_votes = 0;
    for i = 1:rho_length
        for j = 1:theta_length
            if( hough_table(i,j) > max_votes )
                i_index(m) = i;
                j_index(m) = j;
                max_votes = hough_table(i,j);
            end
        end
    end
    
    rho(m) = rho_in(i_index(m));
    theta(m) = theta_in(j_index(m));
    hough_table(i_index(m),j_index(m)) = 0;
    m = m + 1;
    
end


% Effectively generate a small Hough table which contains only values of
%   interest for the validation gate application

rbinv = [0:(2*eps_rho):max(rows, cols)];  % Rho bins for vertical lines
nbinsv = length(rbinv);  % Number of rho bins for vertical lines
ravgv = zeros(1,nbinsv);  % Average rho values for each bin (note that the average value will generally differ slightly than the bin value)
tavgv = zeros(1,nbinsv);  % Average theta values for each bin
vbinv = zeros(1,nbinsv);  % Votes bins for vertical lines

rbinh = [0:(2*eps_rho):max(rows, cols)];
nbinsh = length(rbinh);
ravgh = zeros(1,nbinsh);
tavgh = zeros(1,nbinsh);
vbinh = zeros(1,nbinsh);

% Allow vertical lines along the left side of the image
rbinv(1) = 1;
rbinh(1) = 1;

for i = 1:max_num_lines
    
    % Consider only lines that are either vertical or horizontal, within
    %   tolerance
    condition1 = ( abs(theta(i) - pi/2) <= eps_theta || abs(theta(i) + pi/2) <= eps_theta );  % Horizontal line
    condition2 = ( abs(theta(i) - 0) <= eps_theta );  % Vertical line
    
    if(condition2 && ~( rho(i) == 0 && theta(i) == 0 ))  % Analyze vertical lines (ignore lines exactly along the left side of the image)
        
        for b = 1:nbinsv
            
            % Place each rho value into a bin
            if( abs(rho(i) - rbinv(b)) <= eps_rho )
                ravgv(b) = ravgv(b) + rho(i);
                tavgv(b) = tavgv(b) + theta(i);
                vbinv(b) = vbinv(b) + 1;
                break;
            end
            
        end
        
    elseif(condition1)  % Analyze horizontal lines
        
        if( theta(i) < 0 )
            theta(i) = theta(i) + pi;
            rho(i) = -rho(i);
        end
        
        for b = 1:nbinsh
            
            % Place each rho value into a bin
            if( abs(rho(i) - rbinh(b)) <= eps_rho )
                ravgh(b) = ravgh(b) + rho(i);
                tavgh(b) = tavgh(b) + theta(i);
                vbinh(b) = vbinh(b) + 1;
                break;
            end
            
        end
        
    end
end

% Average the values in ravg and tavg for horizontal and vertical lines
for b = 1:nbinsv
    if( vbinv(b) == 0 )
        ravgv(b) = 0;
        tavgv(b) = 0;
    else
        ravgv(b) = ravgv(b)./vbinv(b);
        tavgv(b) = tavgv(b)./vbinv(b);
    end
end
for b = 1:nbinsh
    if( vbinh(b) == 0 )
        ravgh(b) = 0;
        tavgh(b) = 0;
    else
        ravgh(b) = ravgh(b)./vbinh(b);
        tavgh(b) = tavgh(b)./vbinh(b);
    end
end


%% Extract three lines that fit the criteria for being the validation gate
rmin = 10000;
rmax = -10000;
for b = 1:nbinsv
    
    % Extract the left-most vertical line
    if( ravgv(b) < rmin && ravgv(b) ~= 0 )
        rmin = ravgv(b);
        rho_gate(1) = ravgv(b);
        theta_gate(1) = tavgv(b);
    end
    
    % Extract the right-most vertical line
    if( ravgv(b) > rmax && ravgv(b) ~= 0 )
        rmax = ravgv(b);
        rho_gate(3) = ravgv(b);
        theta_gate(3) = tavgv(b);
    end
    
end

% Check that the distance between the vertical lines is much greater than
%   the minimum expected distance, eps_rho
if( abs(rho_gate(3) - rho_gate(1)) < 2*eps_rho )
    rho_gate(1) = 0;
    rho_gate(3) = 0;
    theta_gate(1) = 0;
    theta_gate(3) = 0;
end

%rmin = 10000;
vmax = 0;
for b = 1:nbinsh
    
    % Extract the horizontal line with the most votes
    if( vbinh(b) > vmax && ravgh(b) ~= 0 )
        vmax = vbinh(b);
        rho_gate(2) = ravgh(b);
        theta_gate(2) = tavgh(b);
    end
    
%    % Extract the horizontal line that is highest up in the image
%    if( ravgh(b) < rmin && ravgh(b) ~= 0 )
%        rmin = ravgh(b);
%        rho_gate(2) = ravgh(b);
%        theta_gate(2) = tavgh(b);
%    end
end


%% Compute targeting information
% Compute intersections
r1 = (  ( rho_gate(1)/cos(theta_gate(1)) ) - ( rho_gate(2)/cos(theta_gate(2)) )  )*(  1/( tan(theta_gate(1)) - tan(theta_gate(2)) )  );
c1 = ( 1/cos(theta_gate(1)) )*( rho_gate(1) - r1*sin(theta_gate(1)) );

r3 = (  ( rho_gate(2)/cos(theta_gate(2)) ) - ( rho_gate(3)/cos(theta_gate(3)) )  )*(  1/( tan(theta_gate(2)) - tan(theta_gate(3)) )  );
c3 = ( 1/cos(theta_gate(2)) )*( rho_gate(2) - r3*sin(theta_gate(2)) );

r2 = (r1 + r3)/2;
c2 = (c1 + c3)/2;

% Compute gate width
w = sqrt( (r3 - r1)^2 + (c3 - c1)^2 );

% Form unit vector pointing downward, parallel to gate posts
tavg = ( theta_gate(1) + (theta_gate(2) - pi/2) + theta_gate(3) )/3;
u = [1 tan(tavg)];
u = u./norm(u);

% Compute target location
th = target_height*gate_aspect_ratio*w;
r_t = r2 + th*u(1);
c_t = c2 + th*u(2);

% Determine if a gate is present (very simple, potentially inaccurate)
if( sum( (rho_gate == 0) + (theta_gate == 0) ) > 0 )
    
    gate_found = 0;
    target_z = 0;
    target_y = 0;
    target_yaw = 0;
    
else
    
    gate_found = 1;
    
    % Transform target r, c to global coordinate system
    target_z = r_t - floor(rows/2);
    target_y = c_t - floor(cols/2);
    target_yaw = Forward_Fov*(target_y/cols);
    
end


return
